simulink library "robot"
libraries: AtomicLibrary x3, BusImpl x1

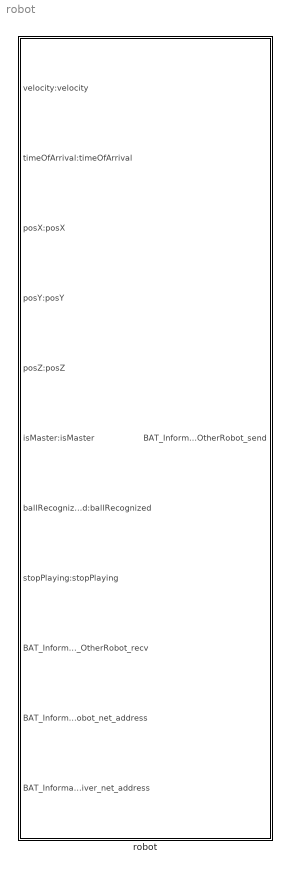
== system robot ==
  robot : Subsystem  Tag=id=_Fl0XEN8LEeKgPPszxxPBOg

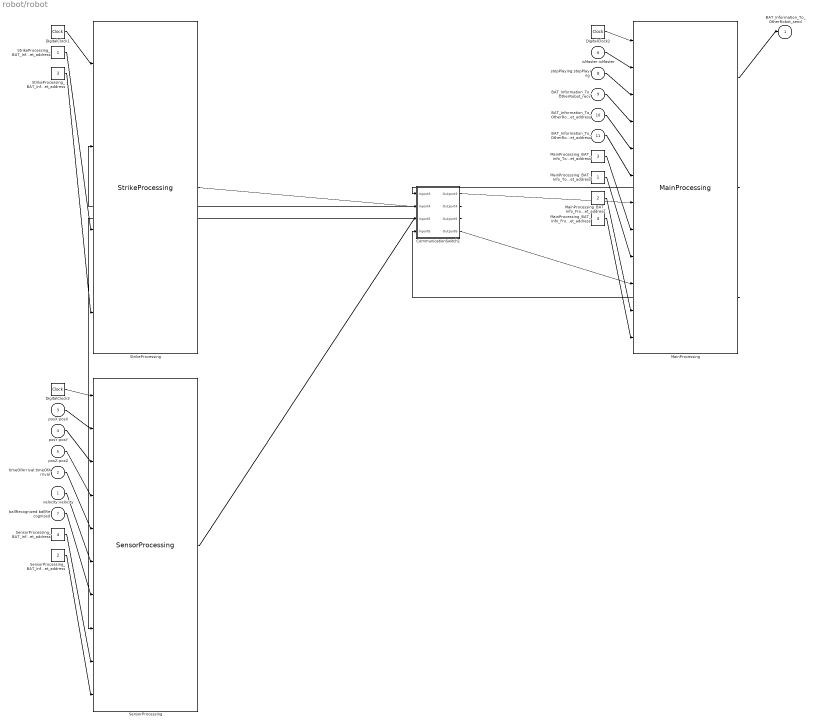
== system robot/robot ==
  velocity:velocity : Inport  Tag=id=_F7lLsN8LEeKgPPszxxPBOg  Port=1  DataType=double  OutDataType=fixdt(1, 16)  OutScaling=2^0  OutDataTypeStr=double
  timeOfArrival:timeOfArrival : Inport  Tag=id=_F7uVoN8LEeKgPPszxxPBOg  Port=2  DataType=double  OutDataType=fixdt(1, 16)  OutScaling=2^0  OutDataTypeStr=double
  posX:posX : Inport  Tag=id=_F7570N8LEeKgPPszxxPBOg  Port=3  DataType=double  OutDataType=fixdt(1, 16)  OutScaling=2^0  OutDataTypeStr=double
  posY:posY : Inport  Tag=id=_F8GwIN8LEeKgPPszxxPBOg  Port=4  DataType=double  OutDataType=fixdt(1, 16)  OutScaling=2^0  OutDataTypeStr=double
  posZ:posZ : Inport  Tag=id=_F8WAsN8LEeKgPPszxxPBOg  Port=5  DataType=double  OutDataType=fixdt(1, 16)  OutScaling=2^0  OutDataTypeStr=double
  isMaster:isMaster : Inport  Tag=id=_F8l4UN8LEeKgPPszxxPBOg  Port=6  DataType=boolean  OutDataType=fixdt(1, 16)  OutScaling=2^0  OutDataTypeStr=boolean
  ballRecognized:ballRecognized : Inport  Tag=id=_F80h0N8LEeKgPPszxxPBOg  Port=7  DataType=boolean  OutDataType=fixdt(1, 16)  OutScaling=2^0  OutDataTypeStr=boolean
  stopPlaying:stopPlaying : Inport  Tag=id=_F9AvEN8LEeKgPPszxxPBOg  Port=8  DataType=boolean  OutDataType=fixdt(1, 16)  OutScaling=2^0  OutDataTypeStr=boolean
  BAT_Information_To_OtherRobot_recv : Inport  Tag=id=_F9bl0N8LEeKgPPszxxPBOg  Port=9  DataType=auto  OutDataType=fixdt(1, 16)  OutScaling=2^0  UseBusObject=on  OutDataTypeStr=Inherit: auto
      settings: BusObject=PacketBus
  BAT_Information_To_OtherRobot_net_address : Inport  Tag=id=_F9cM4d8LEeKgPPszxxPBOg  Port=10  DataType=uint8  OutDataType=fixdt(1, 16)  OutScaling=2^0  OutDataTypeStr=uint8
  BAT_Information_To_OtherRobot_receiver_net_address : Inport  Tag=id=_F9cM4t8LEeKgPPszxxPBOg  Port=11  DataType=uint8  OutDataType=fixdt(1, 16)  OutScaling=2^0  OutDataTypeStr=uint8
  BAT_Information_To_OtherRobot_send : Outport  Tag=id=_F9cM4N8LEeKgPPszxxPBOg  Port=1  DataType=auto  OutDataType=fixdt(1, 16)  OutScaling=2^0  UseBusObject=on  OutDataTypeStr=Inherit: auto
      settings: BusObject=PacketBus
  CommunicationSwitch1 : Subsystem  Tag=id=_Fl0XEd8LEeKgPPszxxPBOg  LoadFcn=MainBusGenerator
  StrikeProcessing : AtomicLibrary/StrikeProcessing  Tag=id=_FmOmwN8LEeKgPPszxxPBOg
  DigitalClock1 : DigitalClock  Tag=id=_FmPN0d8LEeKgPPszxxPBOg  SampleTime=0.001
  MainProcessing : AtomicLibrary/MainProcessing  Tag=id=_FmSRIN8LEeKgPPszxxPBOg
  DigitalClock2 : DigitalClock  Tag=id=_FmS4MN8LEeKgPPszxxPBOg  SampleTime=0.001
  SensorProcessing : AtomicLibrary/SensorProcessing  Tag=id=_FmY-0N8LEeKgPPszxxPBOg
  DigitalClock3 : DigitalClock  Tag=id=_FmZl4d8LEeKgPPszxxPBOg  SampleTime=0.001
  StrikeProcessing_BAT_Info1_net_address : Constant  Tag=id=_F4zkgd8LEeKgPPszxxPBOg  Value=1  OutDataTypeMode=uint8  OutDataTypeStr=uint8
  MainProcessing_BAT_Info_ToStrikeProcessing1_net_address : Constant  Tag=id=_F498kd8LEeKgPPszxxPBOg  Value=3  OutDataTypeMode=uint8  OutDataTypeStr=uint8
  MainProcessing_BAT_Info_From_SensorProcessing1_net_address : Constant  Tag=id=_F5Q3gd8LEeKgPPszxxPBOg  Value=2  OutDataTypeMode=uint8  OutDataTypeStr=uint8
  SensorProcessing_BAT_Info1_net_address : Constant  Tag=id=_F5fhAd8LEeKgPPszxxPBOg  Value=4  OutDataTypeMode=uint8  OutDataTypeStr=uint8
  MainProcessing_BAT_Info_ToStrikeProcessing1_receiver_net_address : Constant  Tag=id=_HBqC9d8LEeKgPPszxxPBOg  Value=1  OutDataTypeMode=uint8  OutDataTypeStr=uint8
  StrikeProcessing_BAT_Info1_receiver_net_address : Constant  Tag=id=_HBqqAd8LEeKgPPszxxPBOg  Value=3  OutDataTypeMode=uint8  OutDataTypeStr=uint8
  SensorProcessing_BAT_Info1_receiver_net_address : Constant  Tag=id=_HBzM498LEeKgPPszxxPBOg  Value=2  OutDataTypeMode=uint8  OutDataTypeStr=uint8
  MainProcessing_BAT_Info_From_SensorProcessing1_receiver_net_address : Constant  Tag=id=_HBzz8d8LEeKgPPszxxPBOg  Value=4  OutDataTypeMode=uint8  OutDataTypeStr=uint8
  wires:
  DigitalClock1/1 -> StrikeProcessing/1
  DigitalClock2/1 -> MainProcessing/1
  DigitalClock3/1 -> SensorProcessing/1
  StrikeProcessing_BAT_Info1_net_address/1 -> StrikeProcessing/3
  MainProcessing_BAT_Info_ToStrikeProcessing1_net_address/1 -> MainProcessing/8
  MainProcessing_BAT_Info_From_SensorProcessing1_net_address/1 -> MainProcessing/11
  SensorProcessing_BAT_Info1_net_address/1 -> SensorProcessing/9
  MainProcessing/2 -> CommunicationSwitch1/1(Inport3)
  StrikeProcessing/1 -> CommunicationSwitch1/2(Inport4)
  CommunicationSwitch1/2(Outport4) -> StrikeProcessing/2
  CommunicationSwitch1/1(Outport3) -> MainProcessing/7
  MainProcessing_BAT_Info_ToStrikeProcessing1_receiver_net_address/1 -> MainProcessing/9
  StrikeProcessing_BAT_Info1_receiver_net_address/1 -> StrikeProcessing/4
  SensorProcessing/1 -> CommunicationSwitch1/3(Inport5)
  MainProcessing/3 -> CommunicationSwitch1/4(Inport6)
  CommunicationSwitch1/4(Outport6) -> MainProcessing/10
  CommunicationSwitch1/3(Outport5) -> SensorProcessing/8
  SensorProcessing_BAT_Info1_receiver_net_address/1 -> SensorProcessing/10
  MainProcessing_BAT_Info_From_SensorProcessing1_receiver_net_address/1 -> MainProcessing/12
  isMaster:isMaster/1 -> MainProcessing/2
  stopPlaying:stopPlaying/1 -> MainProcessing/3
  posY:posY/1 -> SensorProcessing/3
  velocity:velocity/1 -> SensorProcessing/6
  timeOfArrival:timeOfArrival/1 -> SensorProcessing/5
  posZ:posZ/1 -> SensorProcessing/4
  ballRecognized:ballRecognized/1 -> SensorProcessing/7
  posX:posX/1 -> SensorProcessing/2
  BAT_Information_To_OtherRobot_recv/1 -> MainProcessing/4
  MainProcessing/1 -> BAT_Information_To_OtherRobot_send/1
  BAT_Information_To_OtherRobot_receiver_net_address/1 -> MainProcessing/6
  BAT_Information_To_OtherRobot_net_address/1 -> MainProcessing/5

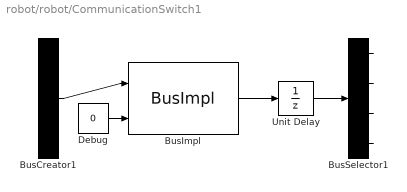
== system robot/robot/CommunicationSwitch1 ==
  Inport3 : Inport  Tag=id=_HBqC8d8LEeKgPPszxxPBOg  Port=1  DataType=auto  OutDataType=fixdt(1, 16)  OutScaling=2^0  UseBusObject=on  OutDataTypeStr=Inherit: auto
      settings: BusObject=PacketBus
  Inport4 : Inport  Tag=id=_HBqC898LEeKgPPszxxPBOg  Port=2  DataType=auto  OutDataType=fixdt(1, 16)  OutScaling=2^0  UseBusObject=on  OutDataTypeStr=Inherit: auto
      settings: BusObject=PacketBus
  Inport5 : Inport  Tag=id=_HByl1d8LEeKgPPszxxPBOg  Port=3  DataType=auto  OutDataType=fixdt(1, 16)  OutScaling=2^0  UseBusObject=on  OutDataTypeStr=Inherit: auto
      settings: BusObject=PacketBus
  Inport6 : Inport  Tag=id=_HBzM4d8LEeKgPPszxxPBOg  Port=4  DataType=auto  OutDataType=fixdt(1, 16)  OutScaling=2^0  UseBusObject=on  OutDataTypeStr=Inherit: auto
      settings: BusObject=PacketBus
  Outport3 : Outport  Tag=id=_HBqC8t8LEeKgPPszxxPBOg  Port=1  DataType=auto  OutDataType=fixdt(1, 16)  OutScaling=2^0  UseBusObject=on  OutDataTypeStr=Inherit: auto
      settings: BusObject=PacketBus
  Outport4 : Outport  Tag=id=_HBqC9N8LEeKgPPszxxPBOg  Port=2  DataType=auto  OutDataType=fixdt(1, 16)  OutScaling=2^0  UseBusObject=on  OutDataTypeStr=Inherit: auto
      settings: BusObject=PacketBus
  Outport5 : Outport  Tag=id=_HBzM4N8LEeKgPPszxxPBOg  Port=3  DataType=auto  OutDataType=fixdt(1, 16)  OutScaling=2^0  UseBusObject=on  OutDataTypeStr=Inherit: auto
      settings: BusObject=PacketBus
  Outport6 : Outport  Tag=id=_HBzM4t8LEeKgPPszxxPBOg  Port=4  DataType=auto  OutDataType=fixdt(1, 16)  OutScaling=2^0  UseBusObject=on  OutDataTypeStr=Inherit: auto
      settings: BusObject=PacketBus
  BusCreator1 : BusCreator  Inputs=4  UseBusObject=on
      settings: BusObject=MainBus
  BusSelector1 : BusSelector  OutputSignals=rc1,rc2,rc3,rc4
  Unit Delay : UnitDelay  SampleTime=-1
  BusImpl : BusImpl/BusImpl
  Debug : Constant  Value=0  OutDataType=fixdt(1, 16)  OutScaling=2^0
  wires:
  BusImpl/1 -> Unit Delay/1
  BusCreator1/1 -> BusImpl/1
  Unit Delay/1 -> BusSelector1/1
  Inport3/1 -> BusCreator1/1  "rc1"
  Inport4/1 -> BusCreator1/2  "rc2"
  Inport5/1 -> BusCreator1/3  "rc3"
  Inport6/1 -> BusCreator1/4  "rc4"
  BusSelector1/1 -> Outport3/1
  BusSelector1/2 -> Outport4/1
  BusSelector1/3 -> Outport5/1
  BusSelector1/4 -> Outport6/1
  Debug/1 -> BusImpl/2
